simulink library "Solar_Collector_basic"  (R2018b)
settings: Solver=ode45  StartTime=0.0  StopTime=10.0  RelTol=1e-3  EnableMultiTasking=on
undefined symbols (not defined in the file): acol, c1, c2, c3, c4, c5, c6, tini
settings Model: Creator=drhf  LastModifiedBy=P41573
settings DataIOCC: LimitDataPoints=on  SaveFormat=Array  SignalLoggingSaveFormat=ModelDataLogs
settings OptimizationCC: ExpressionDepthLimit=2147483647  LifeSpan=inf
settings DebuggingCC: UnderspecifiedInitializationDetection=Classic  MergeDetectMultiDrivingBlocksExec=none  SolverPrmCheckMsg=warning  FcnCallInpInsideContextMsg=warning  StateNameClashWarn=warning  SFUnexpectedBacktrackingDiag=warning  SFNoUnconditionalDefaultTransitionDiag=warning  SFExecutionAtInitializationDiag=none
settings HardwareCC: ProdBitPerPointer=32  ProdBitPerSizeT=32  ProdBitPerPtrDiffT=32  ProdLargestAtomicFloat=None  ProdIntDivRoundTo=Undefined  ProdEndianess=Unspecified  ProdWordSize=32  ProdHWDeviceType=32-bit Generic
settings ModelReferenceCC: PropagateSignalLabelsOutOfModel=off
settings SFSimCC: SimUseLocalCustomCode=off
settings RTWCC: RTWUseLocalCustomCode=off
settings CodeAppCC: StateflowObjectComments=on
settings GRTTargetCC: TargetLangStandard=C89/C90 (ANSI)  GeneratePreprocessorConditionals=Disable all  CombineOutputUpdateFcns=off  GRTInterface=on
settings ConfigComp: CovMetricSettings=dw  CovHtmlReporting=on  CovSaveCumulativeToWorkspaceVar=on  CovSaveSingleToWorkspaceVar=on  CovExternalEMLEnable=off

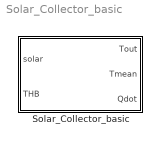
== system Solar_Collector_basic ==
  Solar_Collector_basic : Subsystem  mask(Basic Solar Thermal Collector){acol=acol, c1=c1, c2=c2, c3=c3, c4=c4, c5=c5, c6=c6, tini=tini}
      mask prompts: acol "A : collector surface  [m²]"; c1 "c1 : heat loss coefficient at (Tm-Ta)=0  [W/(m²*K)]"; c2 "c2: temperature dependence of the heat loss coefficient [W/(m*K)²]"; c3 "c3 : wind speed dependence of the heat loss coefficient [J/(m³K)]"; c4 "c4 : sky temperature dependence of the heat loss coefficient [W/(m²K)]"; c5 "c5 : effective thermal capacity [J/(m²K)]"; c6 "c6 : wind dependence in the zero loss efficiency [s/m]"; tini "initial temperature [degree centigrade]"
      mask help: Model according to EN 12975 / ISO 22975
      mask Help: web(fullfile(path_carnot('help'),'Solar_Collector_basic.html'),'-helpbrowser')
      mask Display: disp('solar thermal\ncollector\nEN 12975')

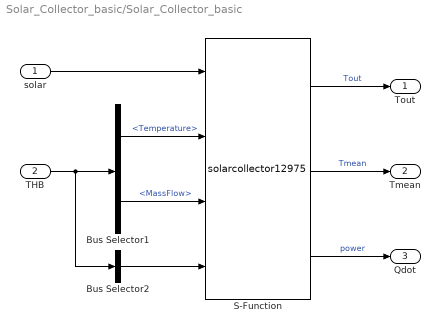
== system Solar_Collector_basic/Solar_Collector_basic ==
  solar : Inport
  THB : Inport  Port=2
  Bus Selector1 : BusSelector  OutputSignals=Temperature,MassFlow
  Bus Selector2 : BusSelector  OutputSignals=Pressure,FluidType,FluidMix  OutputAsBus=on
  S-Function : S-Function  FunctionName=solarcollector12975  Parameters=acol, c1, c2, c3, c4, c5, c6, tini  SFunctionDeploymentMode=off  EnableBusSupport=off
  Tout : Outport
  Tmean : Outport  Port=2
  Qdot : Outport  Port=3
  wires:
  S-Function/3 -> Qdot/1  "power"
  S-Function/2 -> Tmean/1  "Tmean"
  S-Function/1 -> Tout/1  "Tout"
  solar/1 -> S-Function/1
  THB/1 -> Bus Selector2/1, Bus Selector1/1
  Bus Selector2/1 -> S-Function/4
  Bus Selector1/1 -> S-Function/2  "<Temperature>"
  Bus Selector1/2 -> S-Function/3  "<MassFlow>"
